simulink model "scalarcalculator"  (R2021a)
settings: Solver=FixedStepAuto  StartTime=0.0  StopTime=10.0  RelTol=1e-3
libraries: simulink x4
settings Model: Creator=user  LastModifiedBy=user
settings OptimizationCC: DefaultParameterBehavior=Inlined  EnhancedBackFolding=on  PassReuseOutputArgsAs=Individual arguments  ZeroExternalMemoryAtStartup=off  ZeroInternalMemoryAtStartup=off  OptimizeBlockOrder=speed  DifferentSizesBufferReuse=on  OptimizationCustomize=off  EfficientTunableParamExpr=on
settings DebuggingCC: ParameterTunabilityLossMsg=error
settings SFSimCC: MATLABDynamicMemAlloc=off
settings RTWCC: SystemTargetFile=ert.tlc  GenCodeOnly=on  TemplateMakefile=ert_default_tmf  GenerateReport=on  IncludeHyperlinkInReport=on  LaunchReport=on  GenerateTraceInfo=on
settings CodeAppCC: ForceParamTrailComments=on  IgnoreCustomStorageClasses=off  OperatorAnnotations=on  SimulinkDataObjDesc=on  SFDataObjDesc=on  InsertBlockDesc=on
settings ERTTargetCC: TargetLangStandard=C99 (ISO)  GenerateSampleERTMain=on  InlinedParameterPlacement=NonHierarchical  ERTCustomFileTemplate=example_file_process.tlc

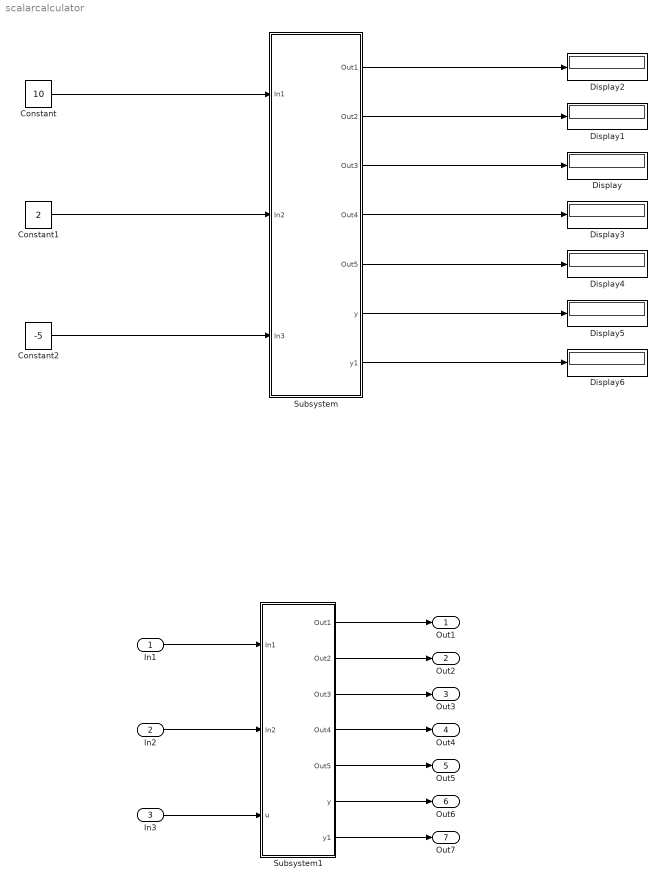
== system scalarcalculator ==
  In1 : Inport
  In2 : Inport  Port=2
  In3 : Inport  Port=3
  Constant : Constant  Value=10
  Constant1 : Constant  Value=2
  Constant2 : Constant  Value=-5
  Display{,1..6} (7 alike) : Display
  Subsystem : Subsystem
  Subsystem1 : Subsystem
  Out1 : Outport
  Out2 : Outport  Port=2
  Out3 : Outport  Port=3
  Out4 : Outport  Port=4
  Out5 : Outport  Port=5
  Out6 : Outport  Port=6
  Out7 : Outport  Port=7
  wires:
  Constant/1 -> Subsystem/1(In1)
  Constant1/1 -> Subsystem/2(In2)
  Constant2/1 -> Subsystem/3(In3)
  Subsystem/1(Out1) -> Display2/1
  Subsystem/2(Out2) -> Display1/1
  Subsystem/3(Out3) -> Display/1
  Subsystem/4(Out4) -> Display3/1
  Subsystem/5(Out5) -> Display4/1
  Subsystem/6(y) -> Display5/1
  Subsystem/7(y1) -> Display6/1
  In1/1 -> Subsystem1/1(In1)
  In2/1 -> Subsystem1/2(In2)
  In3/1 -> Subsystem1/3(u)
  Subsystem1/1(Out1) -> Out1/1
  Subsystem1/2(Out2) -> Out2/1
  Subsystem1/3(Out3) -> Out3/1
  Subsystem1/4(Out4) -> Out4/1
  Subsystem1/5(Out5) -> Out5/1
  Subsystem1/6(y) -> Out6/1
  Subsystem1/7(y1) -> Out7/1

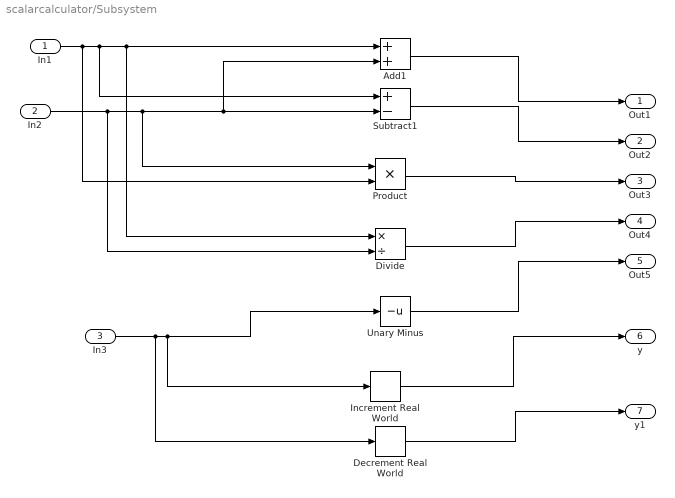
== system scalarcalculator/Subsystem ==
  In1 : Inport
  In2 : Inport  Port=2
  In3 : Inport  Port=3
  Add1 : Sum
  Decrement Real World : simulink/Additional Math & Discrete/Additional Math: Increment - Decrement/Decrement Real World
      settings: SourceProductBaseCode=SL
  Divide : Product  Inputs=*/
  Increment Real World : simulink/Additional Math & Discrete/Additional Math: Increment - Decrement/Increment Real World
      settings: SourceProductBaseCode=SL
  Product : Product
  Subtract1 : Sum  Inputs=+-
  Unary Minus : UnaryMinus
  Out1 : Outport
  Out2 : Outport  Port=2
  Out3 : Outport  Port=3
  Out4 : Outport  Port=4
  Out5 : Outport  Port=5
  y : Outport  Port=6
  y1 : Outport  Port=7
  wires:
  In2/1 -> Divide/2, Product/1, Subtract1/2, Add1/2
  In3/1 -> Decrement Real World/1, Increment Real World/1, Unary Minus/1
  Increment Real World/1 -> y/1
  In1/1 -> Product/2, Subtract1/1, Divide/1, Add1/1
  Subtract1/1 -> Out2/1
  Divide/1 -> Out4/1
  Product/1 -> Out3/1
  Add1/1 -> Out1/1
  Unary Minus/1 -> Out5/1
  Decrement Real World/1 -> y1/1

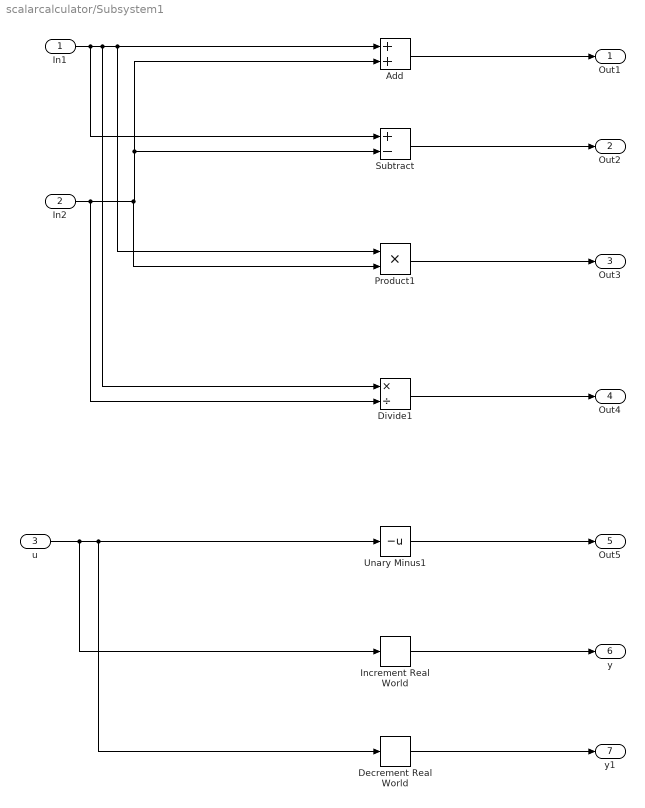
== system scalarcalculator/Subsystem1 ==
  In1 : Inport
  In2 : Inport  Port=2
  u : Inport  Port=3
  Add : Sum
  Decrement Real World : simulink/Additional Math & Discrete/Additional Math: Increment - Decrement/Decrement Real World
      settings: SourceProductBaseCode=SL
  Divide1 : Product  Inputs=*/
  Increment Real World : simulink/Additional Math & Discrete/Additional Math: Increment - Decrement/Increment Real World
      settings: SourceProductBaseCode=SL
  Product1 : Product
  Subtract : Sum  Inputs=+-
  Unary Minus1 : UnaryMinus
  Out1 : Outport
  Out2 : Outport  Port=2
  Out3 : Outport  Port=3
  Out4 : Outport  Port=4
  Out5 : Outport  Port=5
  y : Outport  Port=6
  y1 : Outport  Port=7
  wires:
  In1/1 -> Subtract/1, Divide1/1, Product1/1, Add/1
  u/1 -> Increment Real World/1, Decrement Real World/1, Unary Minus1/1
  Unary Minus1/1 -> Out5/1
  In2/1 -> Divide1/2, Product1/2, Subtract/2, Add/2
  Increment Real World/1 -> y/1
  Subtract/1 -> Out2/1
  Product1/1 -> Out3/1
  Decrement Real World/1 -> y1/1
  Divide1/1 -> Out4/1
  Add/1 -> Out1/1
